simulink model "Proof_instability"  (R2025a)
settings: Solver=VariableStepAuto  StartTime=0.0  StopTime=10  RelTol=1e-3
settings Model: Creator=Faheem  LastModifiedBy=Faheem

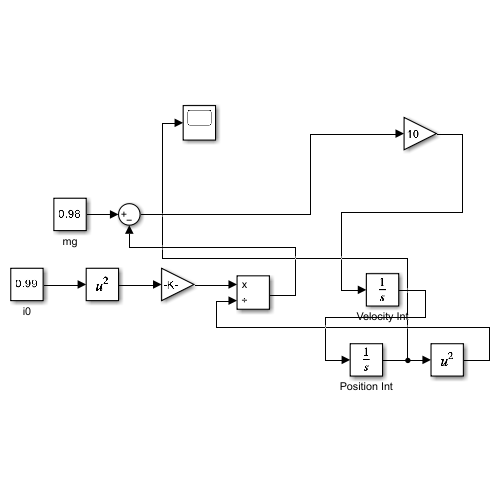
[thumbnail: Simulink's stored preview of the top-level diagram]
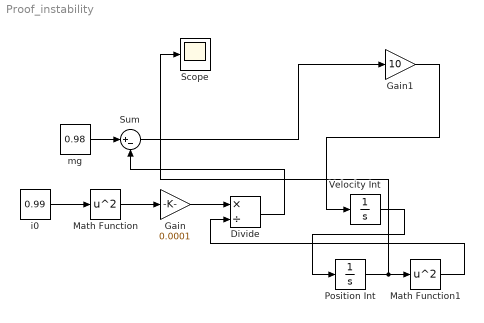
== system Proof_instability ==
  Divide : Product  Inputs=*/
  Gain : Gain  Gain=0.0001
  Gain1 : Gain  Gain=10
  Math Function : Math  Operator=square
  Math Function1 : Math  Operator=square
  Position Int : Integrator  InitialCondition=.0101
  Scope : Scope
      settings: ActiveDisplayYMinimum=-16.692616605952828  ActiveDisplayYMaximum=111.97156604289947
  Sum : Sum  Inputs=|+-
  Velocity Int : Integrator
  i0 : Constant  Value=0.99
  mg : Constant  Value=0.98
  wires:
  i0/1 -> Math Function/1
  Math Function/1 -> Gain/1
  Gain/1 -> Divide/1
  Position Int/1 -> Scope/1, Math Function1/1
  Math Function1/1 -> Divide/2
  Divide/1 -> Sum/2
  mg/1 -> Sum/1
  Sum/1 -> Gain1/1
  Gain1/1 -> Velocity Int/1
  Velocity Int/1 -> Position Int/1
